simulink model "unicycle1"  (R2019b)
settings: Solver=VariableStepAuto  StartTime=0.0  StopTime=20  RelTol=1e-3
values from neighbouring files (symbols this model uses):
  A = [0 1 0 0; 68747/250 0 -29463/250 0; 0 0 0 1;-19642/125 0 9821/125 0]    [test_2.m]    (also in test_3.m = [0 1 0 0; 35856471/2703500 0 -2857911/1081400 0; 0 0 0 1;-98; test_4.m = subs(jacobian(x1, x),[te,te1,a,a1,OA,AB,mB,g],x_equi); test_5.m = [0 1 0 0; 9821/750 0 -9821/2250 0; 0 0 0 1;0 0 9821/375 0]; unicycle.m = [0 1 0 0; 0 0 0 0; 0 0 0 1;0 0 5588149/150160 0])
  B = [0; -16/15; 0; 16/15]    [test_2.m]    (also in test_3.m = [0; -2250/5407; 0; 6925/5407]; test_4.m = subs(jacobian(x1, sym('M')),[te,te1,a,a1,OA,AB,mB,g],x_equi); test_5.m = [0;  -8/15; 0; 8/5]; unicycle.m = [0;  6250/17; 0; -12500/1877])
  K = place(A,B,eigs)    [test_2.m]    (also in test_3.m; test_4.m; unicycle.m = acker(A,B,eigs); unicycle_fro.m = place(A,B,eigs1))
libraries: simulink x1
settings Model: Creator=DooDooDude  LastModifiedBy=DooDooDude

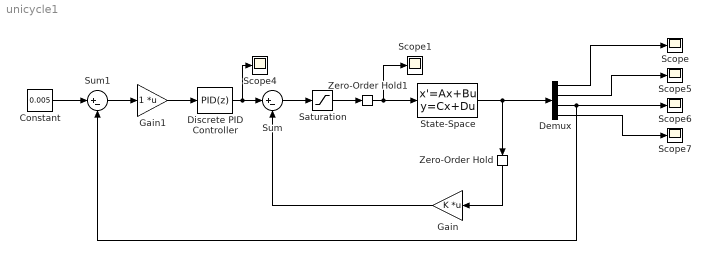
== system unicycle1 ==
  Constant : Constant  Value=0.005
  Demux : Demux
  Discrete PID Controller : simulink/Continuous/PID Controller  Controller=PID  Form=Parallel  TimeDomain=Discrete-time  SampleTime=0.005  IntegratorMethod=Forward Euler  FilterMethod=Forward Euler  ControllerParametersSource=internal  P=1  I=0  D=1  UseFilter=off  N=100  TunerSelectOption=Transfer Function Based (PID Tuner App)  InitialConditionSource=internal  InitialConditionForIntegrator=0  InitialConditionForFilter=0  DifferentiatorICPrevScaledInput=0  ExternalReset=none  TrackingMode=off  Kt=1  LimitOutput=off  UpperSaturationLimit=inf  LowerSaturationLimit=-inf  LinearizeAsGain=off  AntiWindupMode=none  Kb=1  POutMin=[]  POutMax=[]  IOutMin=[]  IOutMax=[]  DOutMin=[]  DOutMax=[]  NOutMin=[]  NOutMax=[]  SumOutMin=[]  SumOutMax=[]  SaturationOutMin=[]  SaturationOutMax=[]  PParamMin=[]  PParamMax=[]  IParamMin=[]  IParamMax=[]  DParamMin=[]  DParamMax=[]  NParamMin=[]  NParamMax=[]  KbParamMin=[]  KbParamMax=[]  KtParamMin=[]  KtParamMax=[]  KbOutMin=[]  KbOutMax=[]  KtOutMin=[]  KtOutMax=[]  IntegratorOutMin=[]  IntegratorOutMax=[]  FilterOutMin=[]  FilterOutMax=[]  SumI1OutMin=[]  SumI1OutMax=[]  SumI2OutMin=[]  SumI2OutMax=[]  SumI3OutMin=[]  SumI3OutMax=[]  SumI4OutMin=[]  SumI4OutMax=[]  SumDOutMin=[]  SumDOutMax=[]  DifferentiatorOutMin=[]  DifferentiatorOutMax=[]  FilterDiffOutCoefMin=[]  FilterDiffOutCoefMax=[]  ReciprocalOutMin=[]  ReciprocalOutMax=[]  SumDenOutMin=[]  SumDenOutMax=[]  SumNumOutMin=[]  SumNumOutMax=[]  DivideOutMin=[]  DivideOutMax=[]  IntegratorContinuousStateAttributes=''  IntegratorStateMustResolveToSignalObject=off  IntegratorRTWStateStorageClass=Auto  FilterContinuousStateAttributes=''  FilterStateMustResolveToSignalObject=off  FilterRTWStateStorageClass=Auto  ParallelPVariant=InternalParameters  IdealPVariant=Disabled  IVariant=InternalParameters  DVariant=InternalParameters  IntegratorVariant=Discrete  SatVariant=Disabled  AWVariant=Passthrough  PCopyVariant=Disabled  TRVariant=Disabled  FdbkBlocksVariant=Forward  IdealPFdbkVariant=Disabled  SatFdbkVariant=Disabled  DerivativeFilterVariant=Differentiator  NVariant=Passthrough  NCopyVariant=Disabled_SignalSpec  FilterICVariant=InternalICsDifferentiator  IntegratorICVariant=InternalICs  ExternalResetVariant=Disabled  TRSumVariant=Passthrough  SumFdbkVariant=Disabled  SumVariant=Sum_PID
  Gain : Gain  Gain=K  Multiplication=Matrix(K*u)
  Gain1 : Gain  Multiplication=Matrix(K*u)
  Saturation : Saturate  UpperLimit=1000  LowerLimit=-1000
  Scope{,1,4..7} (6 alike) : Scope
  State-Space : StateSpace  A=A  B=B  C=eye(4)  D=[0; 0; 0; 0]  InitialCondition=[0; 0; 0; 0]
  Sum : Sum  Inputs=|+-  InputSameDT=on
  Sum1 : Sum  Inputs=|+-  InputSameDT=on
  Zero-Order Hold : ZeroOrderHold  SampleTime=0.005
  Zero-Order Hold1 : ZeroOrderHold  SampleTime=0.005
  wires:
  Gain/1 -> Sum/2
  Zero-Order Hold1/1 -> Scope1/1, State-Space/1
  Saturation/1 -> Zero-Order Hold1/1
  Sum/1 -> Saturation/1
  Constant/1 -> Sum1/1
  Zero-Order Hold/1 -> Gain/1
  Gain1/1 -> Discrete PID Controller/1
  Sum1/1 -> Gain1/1
  Discrete PID Controller/1 -> Scope4/1, Sum/1
  State-Space/1 -> Demux/1, Zero-Order Hold/1
  Demux/1 -> Scope/1
  Demux/2 -> Scope5/1
  Demux/3 -> Sum1/2, Scope6/1
  Demux/4 -> Scope7/1
